simulink model "wirkungsplan"  (R2013b)
settings: Solver=ode45  StartTime=0.0  StopTime=10.0  RelTol=1e-3
values from neighbouring files (symbols this model uses):
  AL = 5e-1    (= 0.5)    [wirkungsplan.m]
  AT = 154    [wirkungsplan.m]
  AV = 5e-1    (= 0.5)    [wirkungsplan.m]
  g = 981    [wirkungsplan.m]
settings Model: Creator=daniw  LastModifiedBy=daniw

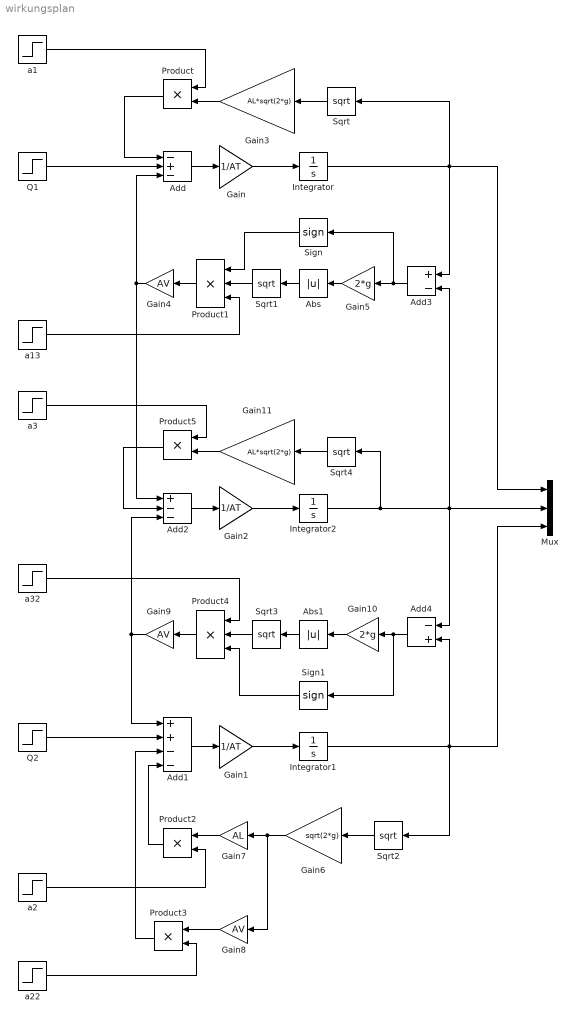
== system wirkungsplan ==
  Abs : Abs
  Abs1 : Abs
  Add : Sum  Inputs=-+-
  Add1 : Sum  Inputs=++--
  Add2 : Sum  Inputs=+--
  Add3 : Sum  Inputs=+-
  Add4 : Sum  Inputs=-+
  Gain : Gain  Gain=1/AT
  Gain1 : Gain  Gain=1/AT
  Gain10 : Gain  Gain=2*g
  Gain11 : Gain  Gain=AL*sqrt(2*g)
  Gain2 : Gain  Gain=1/AT
  Gain3 : Gain  Gain=AL*sqrt(2*g)
  Gain4 : Gain  Gain=AV
  Gain5 : Gain  Gain=2*g
  Gain6 : Gain  Gain=sqrt(2*g)
  Gain7 : Gain  Gain=AL
  Gain8 : Gain  Gain=AV
  Gain9 : Gain  Gain=AV
  Integrator : Integrator
  Integrator1 : Integrator
  Integrator2 : Integrator
  Mux : Mux  Inputs=3
  Product{,2..3,5} (4 alike) : Product
  Product1 : Product  Inputs=3
  Product4 : Product  Inputs=3
  Q1 : Step  SampleTime=0
  Q2 : Step  SampleTime=0
  Sign : Signum
  Sign1 : Signum
  Sqrt{,1..4} (5 alike) : Sqrt  SaturateOnIntegerOverflow=on
  a{1..3,13,22,32} (6 alike) : Step  SampleTime=0
  wires:
  Q1/1 -> Add/2
  Add/1 -> Gain/1
  Gain/1 -> Integrator/1
  Q2/1 -> Add1/2
  Add1/1 -> Gain1/1
  Gain1/1 -> Integrator1/1
  Add2/1 -> Gain2/1
  Gain2/1 -> Integrator2/1
  Product/1 -> Add/1
  Gain3/1 -> Product/2
  Sqrt/1 -> Gain3/1
  Integrator/1 -> Add3/1, Mux/1, Sqrt/1
  a1/1 -> Product/1
  Product1/1 -> Gain4/1
  Gain4/1 -> Add2/1, Add/3
  a13/1 -> Product1/3
  Sign/1 -> Product1/1
  Integrator2/1 -> Sqrt4/1, Mux/2, Add3/2, Add4/1
  Add3/1 -> Gain5/1, Sign/1
  Gain5/1 -> Abs/1
  Abs/1 -> Sqrt1/1
  Sqrt1/1 -> Product1/2
  Integrator1/1 -> Add4/2, Mux/3, Sqrt2/1
  Sqrt2/1 -> Gain6/1
  a2/1 -> Product2/2
  Gain6/1 -> Gain8/1, Gain7/1
  Gain7/1 -> Product2/1
  Gain8/1 -> Product3/1
  a22/1 -> Product3/2
  Product2/1 -> Add1/4
  Product3/1 -> Add1/3
  Product4/1 -> Gain9/1
  Sign1/1 -> Product4/3
  Add4/1 -> Sign1/1, Gain10/1
  Gain10/1 -> Abs1/1
  Abs1/1 -> Sqrt3/1
  Sqrt3/1 -> Product4/2
  Gain9/1 -> Add1/1, Add2/3
  a32/1 -> Product4/1
  Gain11/1 -> Product5/2
  Sqrt4/1 -> Gain11/1
  a3/1 -> Product5/1
  Product5/1 -> Add2/2
